simulink model "Properties_Actuator_Primitives"  (R2012b)
settings: Solver=FixedStepDiscrete  StartTime=0.0  StopTime=10.0  FixedStep=0.1  RelTol=1e-3
settings Model: Creator=Kerianne  LastModifiedBy=Kerianne
settings DataIOCC: SaveFormat=Structure
settings OptimizationCC: InlineParams=on

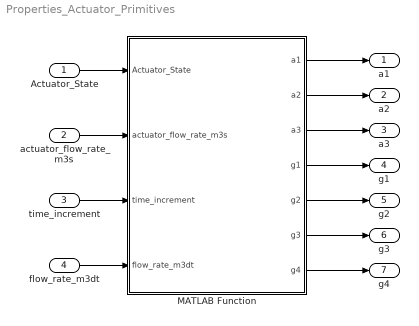
== system Properties_Actuator_Primitives ==
  Actuator_State : Inport  OutDataTypeStr=double
  actuator_flow_rate_m3s : Inport  Port=2  OutDataTypeStr=double
  time_increment : Inport  Port=3  OutDataTypeStr=double
  flow_rate_m3dt : Inport  Port=4  OutDataTypeStr=double
  MATLAB Function : MATLAB Function  TreatAsAtomicUnit=on
  a1 : Outport
  a2 : Outport  Port=2
  a3 : Outport  Port=3
  g1 : Outport  Port=4
  g2 : Outport  Port=5
  g3 : Outport  Port=6
  g4 : Outport  Port=7
  wires:
  Actuator_State/1 -> MATLAB Function/1(Actuator_State)
  actuator_flow_rate_m3s/1 -> MATLAB Function/2(actuator_flow_rate_m3s)
  time_increment/1 -> MATLAB Function/3(time_increment)
  flow_rate_m3dt/1 -> MATLAB Function/4(flow_rate_m3dt)
  MATLAB Function/1(a1) -> a1/1
  MATLAB Function/2(a2) -> a2/1
  MATLAB Function/3(a3) -> a3/1
  MATLAB Function/4(g1) -> g1/1
  MATLAB Function/5(g2) -> g2/1
  MATLAB Function/6(g3) -> g3/1
  MATLAB Function/7(g4) -> g4/1

== matlab function Properties_Actuator_Primitives/MATLAB Function ==
  data: a1 output; a2 output; a3 output; Actuator_State input; g1 output; actuator_flow_rate_m3s input; time_increment input; flow_rate_m3dt input; g2 output; g3 output; g4 output
function [a1, a2, a3, g1, g2, g3, g4]  = verification_condition(Actuator_State, actuator_flow_rate_m3s, time_increment, flow_rate_m3dt)
% Updated 12/23/2014 based on AADL update from 12/02/2014 

% Assumptions
% a1 "The actuator state is either 0 or 1" 
a1 = (Actuator_State == 0 | Actuator_State == 1);
% a2 "The time increment is positive"
a2 = time_increment > 0.0;
% a3 "The actuator flow rate is positive"
a3 = actuator_flow_rate_m3s > 0.0;

%Guarantees
% g1 "If the actuator is receiving an ON|OPEN signal then the flow through the actuator is the max flow rate" 
g1 = actuator_on_cond(Actuator_State, actuator_flow_rate_m3s,time_increment,flow_rate_m3dt);
% g2 "If the actuator is receiving an OFF|CLOSED signal then the flow rate through the actuator is 0.0"
g2 = actuator_off_cond(Actuator_State, flow_rate_m3dt);
% g3 "If there is flow through the actuator, then the actuator is receiving an ON|OPEN signal"
g3 = max_flow_actuator_state(Actuator_State, actuator_flow_rate_m3s,time_increment,flow_rate_m3dt);
% g4 "If the flow is 0.0, then the pump is receiving on OFF|CLOSED signal"
g4 = zero_flow_actuator_state(Actuator_State, flow_rate_m3dt);
	
function c = implies(a,b)      
     c = ((not (a)) || b);
%g1
function result = actuator_on_cond(Actuator_State, actuator_flow_rate_m3s,time_increment,flow_rate_m3dt) 
    UnderThisCondition = (Actuator_State == 1);
    ResultShouldBe = (flow_rate_m3dt == actuator_flow_rate_m3s*time_increment);
    result = implies(UnderThisCondition, ResultShouldBe); 
% g2
function result = actuator_off_cond(Actuator_State, flow_rate_m3dt) 
    UnderThisCondition = (Actuator_State == 0);
    ResultShouldBe = (flow_rate_m3dt == 0.0);
    result = implies(UnderThisCondition, ResultShouldBe);
% g3    
function result = max_flow_actuator_state(Actuator_State, actuator_flow_rate_m3s,time_increment,flow_rate_m3dt) 
    UnderThisCondition = (flow_rate_m3dt == actuator_flow_rate_m3s*time_increment);
    ResultShouldBe = (Actuator_State == 1);
    result = implies(UnderThisCondition, ResultShouldBe); 
% g4    
function result = zero_flow_actuator_state(Actuator_State, flow_rate_m3dt) 
    UnderThisCondition = (flow_rate_m3dt == 0);
    ResultShouldBe = (Actuator_State == 0);
    result = implies(UnderThisCondition, ResultShouldBe);
